simulink model "Exp_07_01_01"  (R2012b)
settings: Solver=ode45  StartTime=0.0  StopTime=5  MaxStep=0.2  RelTol=1e-3
settings Model: Creator=Abraham Xiao  LastModifiedBy=Abraham Xiao
settings DataIOCC: Refine=5

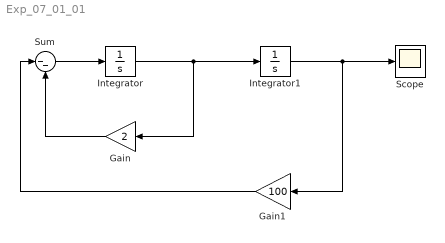
== system Exp_07_01_01 ==
  Gain : Gain  Gain=2
  Gain1 : Gain  Gain=100
  Integrator : Integrator
  Integrator1 : Integrator  InitialCondition=0.05
  Scope : Scope
      settings: TimeRange=5  YMin=-0.06  YMax=0.06
  Sum : Sum  Inputs=|--
  wires:
  Integrator/1 -> Gain/1, Integrator1/1
  Integrator1/1 -> Gain1/1, Scope/1
  Sum/1 -> Integrator/1
  Gain/1 -> Sum/2
  Gain1/1 -> Sum/1
